simulink model "A_Search"  (R2021b)
settings: Solver=ode1  StartTime=0.0  StopTime=Inf  FixedStep=0.020  RelTol=1e-3
libraries: TcTargetLib x8
settings Model: Creator=andre  LastModifiedBy=ATLabor
settings OptimizationCC: DefaultParameterBehavior=Inlined  LocalBlockOutputs=off
settings DebuggingCC: UnconnectedInputMsg=none  UnconnectedOutputMsg=none  UnconnectedLineMsg=none
settings RTWCC: Description=TwinCAT GRT Target  SystemTargetFile=TwinCatGrt.tlc  GenCodeOnly=on  TemplateMakefile=tcgrt_msbuild.tmf  TargetLang=C++  DLArmComputeVersion=20.02.1
settings STFCustomTargetCC: TargetLangStandard=C++11 (ISO)  CombineOutputUpdateFcns=on  CodeInterfacePackaging=Reusable function  CPPClassGenCompliant=on  GRTInterface=off  GenerateAllocFcn=on  SystemTargetFile=TwinCatGrt.tlc
settings GRTTargetCC: TargetLangStandard=C++11 (ISO)  ParMdlRefBuildCompliant=off  CompOptLevelCompliant=off  ConcurrentExecutionCompliant=off  MatFileLogging=off  CodeInterfacePackaging=Reusable function  GenerateAllocFcn=on  UseToolchainInfoCompliant=off  ExtModeMexFile=TcExtModeClient  MultiInstanceErrorCode=Warning

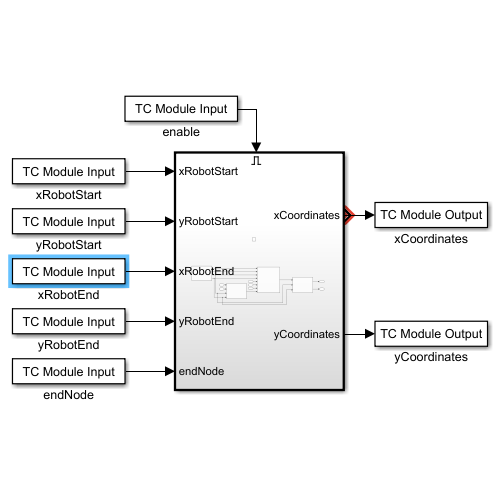
[thumbnail: Simulink's stored preview of the top-level diagram]
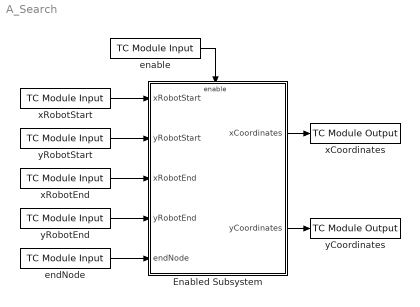
== system A_Search ==
  Enabled Subsystem : Subsystem  TreatAsAtomicUnit=on
  enable : TcTargetLib/TC Module Input  PortDataType=boolean  PortDim=1  Value=0  SampleTime=-1  CodeGenConnectType=DataArea (InputDst)  DataTypeOverride=off
      settings: SourceProductName=Beckhoff TwinCAT Target
  endNode : TcTargetLib/TC Module Input  PortDataType=double  PortDim=1  Value=0  SampleTime=-1  CodeGenConnectType=DataArea (InputDst)  DataTypeOverride=off
      settings: SourceProductName=Beckhoff TwinCAT Target
  xCoordinates : TcTargetLib/TC Module Output  PortDataType=double  PortDim=[101,1]  SampleTime=-1  CodeGenConnectType=DataArea (OutputSrc)  DataTypeOverride=off
      settings: SourceProductName=Beckhoff TwinCAT Target
  xRobotEnd : TcTargetLib/TC Module Input  PortDataType=double  PortDim=1  Value=0  SampleTime=-1  CodeGenConnectType=DataArea (InputDst)  DataTypeOverride=off
      settings: SourceProductName=Beckhoff TwinCAT Target
  xRobotStart : TcTargetLib/TC Module Input  PortDataType=double  PortDim=1  Value=0  SampleTime=-1  CodeGenConnectType=DataArea (InputDst)  DataTypeOverride=off
      settings: SourceProductName=Beckhoff TwinCAT Target
  yCoordinates : TcTargetLib/TC Module Output  PortDataType=double  PortDim=[101,1]  SampleTime=-1  CodeGenConnectType=DataArea (OutputSrc)  DataTypeOverride=off
      settings: SourceProductName=Beckhoff TwinCAT Target
  yRobotEnd : TcTargetLib/TC Module Input  PortDataType=double  PortDim=1  Value=0  SampleTime=-1  CodeGenConnectType=DataArea (InputDst)  DataTypeOverride=off
      settings: SourceProductName=Beckhoff TwinCAT Target
  yRobotStart : TcTargetLib/TC Module Input  PortDataType=double  PortDim=1  Value=0  SampleTime=-1  CodeGenConnectType=DataArea (InputDst)  DataTypeOverride=off
      settings: SourceProductName=Beckhoff TwinCAT Target
  wires:
  enable/1 -> Enabled Subsystem/Enable
  xRobotStart/1 -> Enabled Subsystem/1(xRobotStart)
  yRobotStart/1 -> Enabled Subsystem/2(yRobotStart)
  xRobotEnd/1 -> Enabled Subsystem/3(xRobotEnd)
  yRobotEnd/1 -> Enabled Subsystem/4(yRobotEnd)
  endNode/1 -> Enabled Subsystem/5(endNode)
  Enabled Subsystem/2(yCoordinates) -> yCoordinates/1
  Enabled Subsystem/1(xCoordinates) -> xCoordinates/1

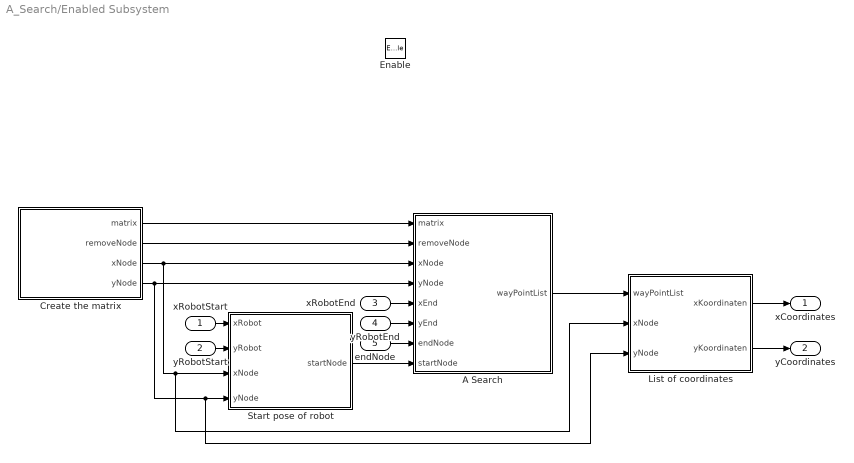
== system A_Search/Enabled Subsystem ==
  xRobotStart : Inport
  yRobotStart : Inport  Port=2
  xRobotEnd : Inport  Port=3
  yRobotEnd : Inport  Port=4
  endNode : Inport  Port=5
  Enable : EnablePort
  " Create the matrix" : MATLAB Function  TreatAsAtomicUnit=on
  A Search : MATLAB Function  TreatAsAtomicUnit=on
  List of coordinates : MATLAB Function  TreatAsAtomicUnit=on
  Start pose of robot : MATLAB Function  TreatAsAtomicUnit=on
  xCoordinates : Outport
  yCoordinates : Outport  Port=2
  wires:
  xRobotStart/1 -> Start pose of robot/1(xRobot)
  yRobotStart/1 -> Start pose of robot/2(yRobot)
  " Create the matrix"/3(xNode) -> A Search/3(xNode), List of coordinates/2(xNode), Start pose of robot/3(xNode)
  " Create the matrix"/4(yNode) -> List of coordinates/3(yNode), Start pose of robot/4(yNode), A Search/4(yNode)
  " Create the matrix"/1(matrix) -> A Search/1(matrix)
  " Create the matrix"/2(removeNode) -> A Search/2(removeNode)
  Start pose of robot/1(startNode) -> A Search/8(startNode)
  xRobotEnd/1 -> A Search/5(xEnd)
  yRobotEnd/1 -> A Search/6(yEnd)
  endNode/1 -> A Search/7(endNode)
  A Search/1(wayPointList) -> List of coordinates/1(wayPointList)
  List of coordinates/1(xKoordinaten) -> xCoordinates/1
  List of coordinates/2(yKoordinaten) -> yCoordinates/1

== matlab function A_Search/Enabled Subsystem/Start pose of robot ==
  data: startNode output double size=1; xRobot input double size=1; yRobot input double size=1; xNode input double size=[144,1]; yNode input double size=[144,1]
function startNode= fcn(xRobot, yRobot, xNode, yNode)

startNode = 0;
startNodeArray = 0;
diff_x = zeros(size(xNode,1),1);
diff_y = zeros(size(yNode,1),1);

for i = 1:size(xNode,1)
    diff_x(i) = abs(xRobot-xNode(i));
end

for i = 1:size(yNode,1)
    diff_y(i) = abs(yRobot-yNode(i));
end

xMin = min(diff_x);
yMin = min(diff_y);

xStart = find(diff_x == xMin);
yStart = find(diff_y == yMin);

startNodeArray = intersect(xStart, yStart);

startNode = startNodeArray(1,1);

== matlab function A_Search/Enabled Subsystem/ Create the matrix ==
  data: matrix output double size=[144,144]; removeNode output double size=[1,12]; xNode output double size=[144,1]; yNode output double size=[144,1]
function [matrix, removeNode, xNode, yNode] = fcn()

numberOfNodes = 144;
numberOfColumns = 18;
matrix = zeros(numberOfNodes);

% Verbindung zu relevanten Knoten
for i = 1:numberOfNodes
    if i-1>0 && mod(i, numberOfColumns) ~= 1
        matrix(i-1,i) = 1000;
    end
    if i+1<numberOfNodes+1 && mod(i,numberOfColumns) ~= 0
        matrix(i+1,i)= 1000;
    end
    if i+numberOfColumns<numberOfNodes+1
        matrix(i+numberOfColumns,i)=1000;
    end
    if i-numberOfColumns>0
        matrix(i-numberOfColumns,i)=1000;
    end
    if i+numberOfColumns+1 < numberOfNodes+1 && mod(i,numberOfColumns) ~= 0
        matrix(i+numberOfColumns+1,i) = sqrt(2)*1000;
    end
    if i+numberOfColumns-1 < numberOfNodes+1 && mod(i, numberOfColumns) ~= 1
        matrix(i+numberOfColumns-1,i) = sqrt(2)*1000;
    end
     if i-numberOfColumns+1 > 0 && mod(i,numberOfColumns) ~= 1
        matrix(i-numberOfColumns+1,i) = sqrt(2)*1000;
    end
    if i-numberOfColumns-1 > 0 && mod(i, numberOfColumns) ~= 0
        matrix(i-numberOfColumns-1,i) = sqrt(2)*1000;
    end
end

% Lösen der Station
removeNode = [93 96 99 102 111 114 117 120 124 125 142 143];
for counter = 1:size(removeNode,2)
    for j = 1:numberOfNodes
        matrix(removeNode(counter),j) = 0;
        matrix(j,removeNode(counter)) = 0;
    end
end

% Umrechung von Knoten in Koordinaten
xNode = zeros(numberOfNodes,1);
yNode = zeros(numberOfNodes,1);
row = 600;
col = 200;
for i = 1:numberOfNodes
    xNode(i) = col;
    yNode(i) = row;
    col = col + 400;
    if mod(i,numberOfColumns) == 0 
        col = 200;
        row = row + 400;
    end 
end

== matlab function A_Search/Enabled Subsystem/A Search ==
  data: matrix input double size=[144,144]; removeNode input double size=[1,12]; xNode input double size=[144,1]; yNode input double size=[144,1]; xEnd input double size=1; yEnd input double size=1; endNode input double size=1; wayPointList output double size=[101,1]; startNode input double size=1
function wayPointList = fcn(matrix, removeNode, xNode, yNode, xEnd, yEnd, endNode, startNode)
numNodes = 144;
openList = zeros(8,5); %1. Node 2. g(x) 3. h(x) 4. f(x) 5. parent node
closedList = zeros(101,5); %1. Node 2. g(x) 3. h(x) 4. f(x) 5. parent node
neighborList = zeros(8,5); %1. Node 2. g(x) 3. h(x) 4. f(x) 5. parent node
step = 1;
index = 1;
overlap = false;
nodefmin = 0;
currentNode = startNode;
parentNode = 0;
noPath = false;
g = 0;
gprev = g;
h = sqrt(power(xNode(startNode)-xEnd,2) + power(yNode(startNode)-yEnd,2));
f = g + h;
fmin = 0;

%Goal reached?
while currentNode ~= endNode
    for counter = 1:size(removeNode,2)
        %The currentnode isn't a hinderance
        if currentNode ~= removeNode(counter)
            noHinderance = true;
        %The currentnode is a hinderance
        else
            noHinderance = false;
            break;
        end
    end
   if noHinderance == true 
        %The smallest f is put in closedlist when 
        closedList(step, 1) = currentNode;
        closedList(step, 2) = g;
        closedList(step, 3) = h;
        closedList(step, 4) = f;
        closedList(step, 5) = parentNode;
        step = step + 1;

        %Clear the openlist and neighborlist
        openList = zeros(8,5);
        neighborList = zeros(8,5);
        index = 1;
    
        %Search the neighbor and put in the neighborlist
        for i = 1:numNodes
            %calculate fowards
            if matrix(currentNode,i) ~= 0
                g = gprev + sqrt(power(xNode(i)-xNode(startNode),2) + power(yNode(i)-yNode(startNode),2));
                h = sqrt(power(xNode(i)-xEnd,2) + power(yNode(i)-yEnd,2));
                neighborList(index,1) = i;
                neighborList(index,2) = g;
                neighborList(index,3) = h;
                neighborList(index,4) = g + h;
                neighborList(index,5) = currentNode;
                index = index + 1;
            end
        end
    
        %the possible neighbors will be inserted in the openlist when it
        %doesn't exist in closedlist
        for i = 1:size(neighborList,1)
            for j = 1:size(closedList,1)
                if neighborList(i) == closedList(j)
                    overlap = true;
                    break;
                end
            end
            if overlap == false
                openList(i,1) = neighborList(i,1);
                openList(i,2) = neighborList(i,2);
                openList(i,3) = neighborList(i,3);
                openList(i,4) = neighborList(i,4);
                openList(i,5) = neighborList(i,5);
            end
            overlap = false;
        end
   else
       openList(nodefmin,:) = [];
   end

    %Search the smallest f in openlist
    flag = false; 
    for i = 1:size(openList,1)
        if openList(i,4) ~= 0
            if flag == false
                fmin = openList(i,4);
                nodefmin = i;
                flag = true;
            end
            if fmin > openList(i,4) 
                fmin = openList(i,4);
                nodefmin = i;
            end   
        end
    end

    %found the smallest f and update the values
    currentNode = openList(nodefmin,1);
    g = openList(nodefmin,2);
    h = openList(nodefmin,3);
    f = openList(nodefmin,4);
    parentNode = openList(nodefmin,5);
    gprev = g;
end

closedList(step, 1) = currentNode;
closedList(step, 2) = g;
closedList(step, 3) = h;
closedList(step, 4) = f;
closedList(step, 5) = parentNode;

wayPointList = zeros(101,1);
for index = 1:step
    wayPointList(index) = closedList(index,1);
end

== matlab function A_Search/Enabled Subsystem/List of coordinates ==
  data: xKoordinaten output double size=[101,1]; wayPointList input double size=[101,1]; xNode input double size=[144,1]; yNode input double size=[144,1]; yKoordinaten output double size=[101,1]
function [xKoordinaten, yKoordinaten]= fcn(wayPointList, xNode, yNode)

sizeList = size(wayPointList,1);
xKoordinaten = zeros(sizeList,1);
yKoordinaten = zeros(sizeList,1);

for i = 1 : sizeList
    if wayPointList(i) ~= 0
        xKoordinaten(i) = xNode(wayPointList(i));
        yKoordinaten(i) = yNode(wayPointList(i));
    end
end
